simulink model "example_microCHPconstant"  (R2016b)
settings: Solver=VariableStepAuto  StartTime=0.0  StopTime=10.0  RelTol=1e-3
libraries: carnot x2
settings Model: Creator=drhf  LastModifiedBy=drhf

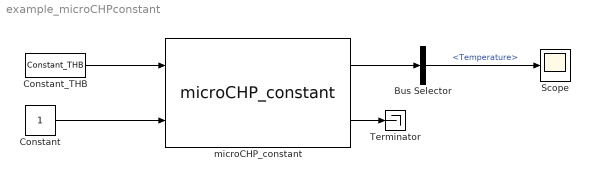
== system example_microCHPconstant ==
  Bus Selector : BusSelector  OutputSignals=Temperature
  Constant : Constant
  Constant_THB : carnot/Source/Simple/Constant_THB  t=40  mdot=0  p=1e5  mID=No Pressure Drop  fluid=Water  mix=0  mix2=0  mix3=0  dia=0.02  hgt=0
  Scope : Scope
  Terminator : Terminator
  microCHP_constant : carnot/Source/Cogeneration/microCHP_constant  P_th=11520  P_el=5500  P_fuel=22030  T_flow_setpoint=80  T_return_max=60
  wires:
  Constant_THB/1 -> microCHP_constant/1
  Constant/1 -> microCHP_constant/2
  microCHP_constant/1 -> Bus Selector/1
  Bus Selector/1 -> Scope/1  "<Temperature>"
  microCHP_constant/2 -> Terminator/1
